simulink library "LIB_NetwokInterface"  (R2016b)
settings: Solver=ode45  StartTime=0.0  StopTime=10.0  RelTol=1e-3  EnableMultiTasking=on
libraries: LIB_NetwokInterface x1
settings Model: Creator=sven  LastModifiedBy=valtin
settings DataIOCC: LimitDataPoints=on  SaveFormat=Array
settings OptimizationCC: LifeSpan=inf
settings DebuggingCC: UnderspecifiedInitializationDetection=Classic  MergeDetectMultiDrivingBlocksExec=none  SolverPrmCheckMsg=warning  StateNameClashWarn=warning  SFUnexpectedBacktrackingDiag=warning  SFNoUnconditionalDefaultTransitionDiag=warning  SFExecutionAtInitializationDiag=none
settings HardwareCC: ProdBitPerPointer=32  ProdBitPerSizeT=32  ProdBitPerPtrDiffT=32  ProdLargestAtomicFloat=None  ProdIntDivRoundTo=Undefined  ProdEndianess=Unspecified  ProdWordSize=32  ProdHWDeviceType=32-bit Generic
settings ModelReferenceCC: PropagateSignalLabelsOutOfModel=off
settings GRTTargetCC: TargetLangStandard=C89/C90 (ANSI)  GeneratePreprocessorConditionals=Disable all
settings ConfigComp: CovMetricSettings=dw  CovHtmlReporting=on  CovSaveCumulativeToWorkspaceVar=on  CovSaveSingleToWorkspaceVar=on  CovExternalEMLEnable=off  CovSFcnEnable=off

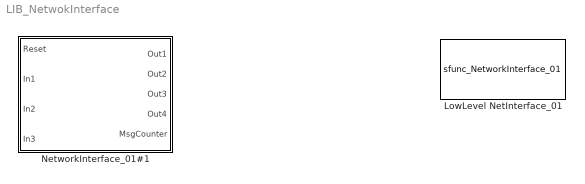
== system LIB_NetwokInterface ==
  LowLevel NetInterface_01 : S-Function  FunctionName=sfunc_NetworkInterface_01  Parameters=numberOfInputs, numberOfOutputs, blockOptions, initialOutputValues, useUDP, startConnection, localPort, remoteIP, remotePort, SampleTime  SFunctionDeploymentMode=off  EnableBusSupport=off  mask(LowLevel NetworkInferface Block){numberOfInputs=5, numberOfOutputs=4, initialOutputValues=0, SampleTime=-1, useUDP=on, startConnection=on, localPort=20000, remoteIP='127.0.0.1', remotePort=20001}
      mask prompts: numberOfInputs "Number of Inputs:"; numberOfOutputs "Number of Outputs:"; initialOutputValues "Initiale Output Values (e.g. 0 or 1 (scaler) or [1,0,1,2]):"; SampleTime "Sample Time:"; useUDP "Use UDP instead of TCP for the connection?"; startConnection "Start the network connection at the start of the Diagramm start?"; localPort "Local Port (Net Input -> Block Output):"; remoteIP "Remote IP (Block Input -> Net Output):"; remotePort "Remote Port (Block Input -> Net Output):"
      mask help: The LowLevel block for the SRT network communication.
      mask init:
      | %% fix numberOfInputs / numberOfOutputs
      | 
      | isInputsZero = 0;
      | isOutputsZero = 0;
      | numberOfInputs  = int32(sum(numberOfInputs));
      | numberOfOutputs = int32(sum(numberOfOutputs));
      | 
      | if (max(size(initialOutputValues)) < numberOfOutputs)
      |     initialOutputValues = ones(1, numberOfOutputs) *initialOutputValues(1);
      | end
      | initialOutputValues = double(initialOutputValues);
      | 
      | if (numberOfInputs <= 0)
      |     numberOfInputs = 1;
      |     isInputsZero = 1;
      | end
      | if (numberOfOutputs <= 0)
      |     numberOfOutputs = 1;
      |     isOutputsZero = 1;
      |     initialOutputValues = double(0);
      | end
      | 
      | useUDP = int32(useUDP);
      | startConnection = int32(startConnection);
      | 
      | localPort = uint32(localPort);
      | remoteIP = [unicode2native(remoteIP, 'ISO-8859-1') 0];
      | remotePort = uint32(remotePort);
      | 
      | blockOptions = [isInputsZero, isOutputsZero];
      | blockOptions = uint32(blockOptions);
      | 
      | %% sfunction parameters
      | % numberOfInputs, numberOfOutputs, blockOptions, initialOutputValues, useUDP, startConnection, localPort, remoteIP, remotePort, sampleTime
      mask Display:
      | % LowLovel NetworkInterface
      | port_label('input',1,'Control');
      | port_label('input',2,'Data');
      | port_label('input',3,'SimTime');
      | 
      | port_label('output',1,'Output');
      | port_label('output',2,'MsgCounter');
  NetworkInterface_01#1 : Subsystem  mask(NetworkInterface Block){inputs=[1,2,1], outputs=[1,2,3,1], initialOutputValues=0, SampleTime=-1, useUDP=on, startConnection=on, localPort=20000, remoteIP='127.0.0.1', remotePort=20001}
      mask prompts: inputs "Define Input Signals (e.g. [1,2,1]):"; outputs "Define Output Signals (e.g. [1,2,1,3]):"; initialOutputValues "Initiale Output Values (e.g. 0 or 1 (scaler) or [1,0,1,2]):"; SampleTime "Sample Time:"; useUDP "Use UDP instead of TCP for the connection?"; startConnection "Start the network connection at the start of the Diagramm start?"; localPort "Local Port (Net Input -> Block Output):"; remoteIP "Remote IP (Block Input -> Net Output):"; remotePort "Remote Port (Block Input -> Net Output):"
      mask help: Network interface block for usage with the SRT.
      mask init:
      | % block initialisation
      | simulink_NetworkInterface_init(gcb, inputs, outputs);
      mask Help:
      | <p><a href="https://github.com/TUB-Control/PaPI/wiki">https://github.com/TUB-Control/PaPI/wiki</a></p>
      | 
      | <h4>This blocks provides following static input signal</h4>
      | 
      | <b>reset</b>: Possible values {0,1}
      | This signal can be used to reset the PaPI Block. The Configuration will be sent again and the current outputs will be to zero.
      | </hr>
      | <h4>This blocks provides following parameters</h4>
      | 
      | <b>[Amount parameters]</b>
      | Used to define the parameters which can be modified in PaPI.
      | [1,2,45] creates two parameters, with size(p1)=1, size(p2)=2, size(p3)=45
      | 
      | <b>[Json Config]</b>
      | Can be used to create Plugins and subcriptions in PaPI.
      | A file name can be used e.g. 'papi_test.json' as well as a file name
      | including its path. It is also possible to directly read the file using
      | the command 'fileread' e.g. fileread('papi_test.json'), but this is not
      | necessary.
      | If no config is used, the input must be (don't forget the single quoation
      | marks at the end and beginning to generate a string, the curly brackets to
      | open and close the Json-Object and don't forget the <b>blank</b> between the curly
      | brackets): '{ }'
      | 
      | <b>[Amount of signals]</b>
      | Defines the amount of input signals which can be subscribed in PaPI
      | 
      | <b>[Local port]</b>
      | <b>[Remote port]</b>
      | <b>[Output size]</b>
      | Defines the maximal vector size which can be sent at a single timestamp.
      | 
      | <b>[Recieve: Msg Length]</b>
      | Defines the maximal vector size which can be recieved at a single timestamp.
      | 
      | <b>[Local IP]</b>
      | <b>[Remote IP]</b>
      mask TypeOptions inputs: LowLevel NetInterface_01/numberOfInputs
      mask Callback inputs:
      | simulinkValueStr = get_param(gcb, 'inputs');
      | if (isempty(simulinkValueStr))
      |     set_param(gcb, 'inputs', '0');
      | else
      |     simulinkValue = evalin('caller', simulinkValueStr);
      |     if (isempty(simulinkValue))
      |         set_param(gcb, 'inputs', '0');
      |     end
      | end
      mask TypeOptions outputs: LowLevel NetInterface_01/numberOfOutputs
      mask Callback outputs:
      | simulinkValueStr = get_param(gcb, 'outputs');
      | if (isempty(simulinkValueStr))
      |     set_param(gcb, 'outputs', '0');
      | else
      |     simulinkValue = evalin('caller', simulinkValueStr);
      |     if (isempty(simulinkValue))
      |         set_param(gcb, 'outputs', '0');
      |     end
      | end
      mask TypeOptions initialOutputValues: LowLevel NetInterface_01/initialOutputValues
      mask TypeOptions SampleTime: Digital Clock/SampleTime | LowLevel NetInterface_01/SampleTime | NetDelay/SampleTime
      mask TypeOptions useUDP: LowLevel NetInterface_01/useUDP
      mask TypeOptions startConnection: LowLevel NetInterface_01/startConnection
      mask TypeOptions localPort: LowLevel NetInterface_01/localPort
      mask TypeOptions remoteIP: LowLevel NetInterface_01/remoteIP
      mask TypeOptions remotePort: LowLevel NetInterface_01/remotePort
      mask Display:
      | %% lables
      | color('blue'); text(0.5, 0.5, 'NetworkInterface','horizontalAlignment','center');
      | 
      | color('black');
      | port_label('input',  1  ,' Control ');
      | 
      | port_label('input', 2, 'IN 1');
      | port_label('input', 3, 'IN 2');
      | port_label('input', 4, 'IN 3');
      | port_label('output', 1, 'OUT 1');
      | port_label('output', 2, 'OUT 2');
      | port_label('output', 3, 'OUT 3');
      | port_label('output', 4, 'OUT 4');
      | port_label('output', 5, 'MsgCounter');

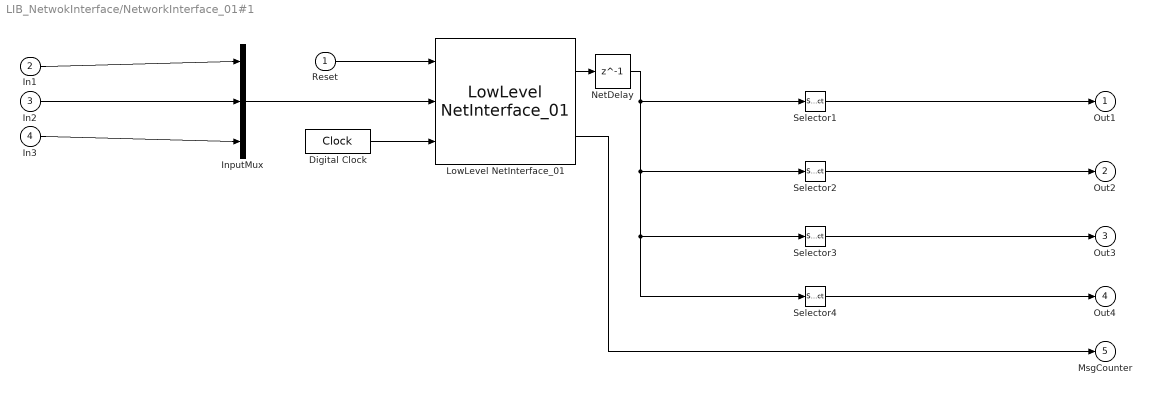
== system LIB_NetwokInterface/NetworkInterface_01#1 ==
  Reset : Inport  PortDimensions=1
  In1 : Inport  Port=2  PortDimensions=1
  In2 : Inport  Port=3  PortDimensions=2
  In3 : Inport  Port=4  PortDimensions=1
  Digital Clock : DigitalClock  SampleTime=SampleTime
  InputMux : Mux  Inputs=3
  LowLevel NetInterface_01 : LIB_NetwokInterface/LowLevel NetInterface_01  numberOfInputs=inputs  numberOfOutputs=outputs  initialOutputValues=initialOutputValues  SampleTime=SampleTime  useUDP=on  startConnection=on  localPort=localPort  remoteIP=remoteIP  remotePort=remotePort
  NetDelay : Delay  DelayLength=1  InitialCondition=0  SampleTime=SampleTime
  Selector1 : Selector  InputPortWidth=7  IndexOptions=Index vector (dialog)  Indices=[1:1]  OutputSizes=1
  Selector2 : Selector  InputPortWidth=7  IndexOptions=Index vector (dialog)  Indices=[2:3]  OutputSizes=1
  Selector3 : Selector  InputPortWidth=7  IndexOptions=Index vector (dialog)  Indices=[4:6]  OutputSizes=1
  Selector4 : Selector  InputPortWidth=7  IndexOptions=Index vector (dialog)  Indices=[7:7]  OutputSizes=1
  Out1 : Outport
  Out2 : Outport  Port=2
  Out3 : Outport  Port=3
  Out4 : Outport  Port=4
  MsgCounter : Outport  Port=5
  wires:
  Digital Clock/1 -> LowLevel NetInterface_01/3
  Selector1/1 -> Out1/1
  Selector2/1 -> Out2/1
  Selector3/1 -> Out3/1
  LowLevel NetInterface_01/1 -> NetDelay/1
  Reset/1 -> LowLevel NetInterface_01/1
  NetDelay/1 -> Selector2/1, Selector3/1, Selector4/1, Selector1/1
  Selector4/1 -> Out4/1
  LowLevel NetInterface_01/2 -> MsgCounter/1
  InputMux/1 -> LowLevel NetInterface_01/2
  In1/1 -> InputMux/1
  In2/1 -> InputMux/2
  In3/1 -> InputMux/3
